simulink model "QuadrotorFinalProjectv4"  (R2018b)
settings: Solver=VariableStepAuto  StartTime=0.0  StopTime=25  RelTol=1e-3
undefined symbols (not defined in the file or in its folder): sigbuilder_block, X, Y, Z
libraries: sm_lib x94, nesl_utility x48, simulink x4
(part 3 of 3)

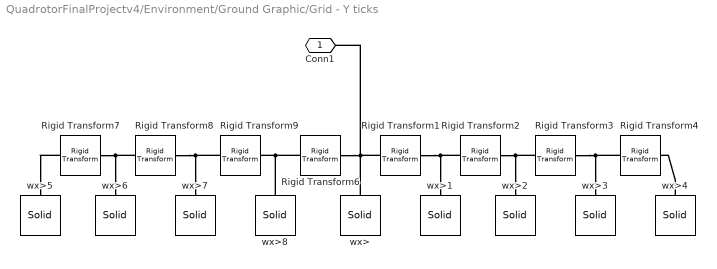
== system QuadrotorFinalProjectv4/Environment/Ground Graphic/Grid - Y ticks ==
  Rigid Transform{1..4,6..9} (8 alike) : sm_lib/Frames and Transforms/Rigid Transform  TranslationMethod=Cartesian  TranslationStandardOffset=0  TranslationLengthUnit=m  TranslationStandardAxis=+Z  TranslationCartesianOffset=[0 10 0]  TranslationROffset=0  TranslationROffsetUnits=m  TranslationZOffset=0  TranslationZOffsetUnits=m  TranslationThetaOffset=0  TranslationThetaOffsetUnits=deg  RotationMethod=None  RotationAngleUnits=deg  RotationStandardAxis=+Z  RotationAngle=0.0  RotationArbitraryAxis=[0 0 1]  FollAlignAxisA=+X  BaseAlignAxisA=+Y  FollAlignAxisB=+Y  BaseAlignAxisB=+Z  RotationSequenceAxes=FollowerAxes  RotationSequence=XYX  RotationSequenceAngles=[0 0 0]  RotationSequenceAnglesUnits=deg  RotationMatrix=[1 0 0; 0 1 0; 0 0 1]
  wx>{,1..8} (9 alike) : sm_lib/Body Elements/Solid  InertiaType=CalculateFromGeometry  Mass=1.6  MassUnits=kg  CenterOfMass=[0 0 0]  CenterOfMassUnits=m  MomentsOfInertia=[1 1 1]  MomentsOfInertiaUnits=kg*m^2  ProductsOfInertia=[0 0 0]  ProductsOfInertiaUnits=kg*m^2  BasedOnType=Mass  Density=1000  DensityUnits=kg/m^3  DoExposeReferenceFrame=on  SerializedFrames=<Frames/>  GraphicType=FromGeometry  MarkerShape=Frame  MarkerSize=10  GraphicVisPropType=SimpleVisualProperties  GraphicDiffuseColor=[1 1 1]  GraphicSpecularColor=[0.5 0.5 0.5 1.0]  GraphicAmbientColor=[0.15 0.15 0.15 1.0]  GraphicEmissiveColor=[0.0 0.0 0.0 1.0]  GraphicShininess=75  GraphicOpacity=0.9  GeometryShape=Brick  RectangleSize=[1 1]  RectangleSizeUnits=m  BrickDimensions=[100 1 0.12]  BrickDimensionUnits=m  CylinderRadius=1  CylinderRadiusUnits=m  CylinderLength=1  CylinderLengthUnits=m  SphereRadius=0.05  SphereRadiusUnits=m  EllipsoidRadii=[1 1 1]  EllipsoidRadiiUnits=m  ExtrusionCrossSection=[1 1; -1 1; -1 -1; 1 -1]  ExtrusionCrossSectionUnits=m  ExtrusionLength=1  ExtrusionLengthUnits=m  PolygonNumSides=3  PolygonOuterRadius=1  PolygonOuterRadiusUnits=m  ExtGeomFileType=STEP  ExtGeomFileUnits=m  RevolutionCrossSection=[1 1; 1 -1; 2 -1; 2 1]  RevolutionCrossSectionUnits=m  RevolutionExtent=Full  RevolutionAngle=180  RevolutionAngleUnits=deg
  Conn1 : PMIOPort  Side=Left
  connections:
  wx>/RConn1 -- Conn1/RConn1 -- Rigid Transform1/LConn1 -- Rigid Transform6/RConn1
  Rigid Transform2/LConn1 -- Rigid Transform1/RConn1 -- wx>1/RConn1
  Rigid Transform2/RConn1 -- Rigid Transform3/LConn1 -- wx>2/RConn1
  wx>8/RConn1 -- Rigid Transform6/LConn1 -- Rigid Transform9/RConn1
  wx>4/RConn1 -- Rigid Transform4/RConn1
  Rigid Transform7/RConn1 -- Rigid Transform8/LConn1 -- wx>6/RConn1
  Rigid Transform7/LConn1 -- wx>5/RConn1
  Rigid Transform3/RConn1 -- wx>3/RConn1 -- Rigid Transform4/LConn1
  Rigid Transform8/RConn1 -- Rigid Transform9/LConn1 -- wx>7/RConn1

== matlab function QuadrotorFinalProjectv4/Quadrotor/SmallSphere1Drag/MATLAB Function1 ==
  data: vx input; y output; vy input; vz input
function y = drag(vx,vy,vz)
radius = 0.02;
y = [-((1/2)*(1)*pi*(radius^(2))*(0.5)*(abs(vx))*vx); ...
    -((1/2)*(1)*pi*(radius^(2))*(0.5)*(abs(vy))*vy); ...
    -((1/2)*(1)*pi*(radius^(2))*(0.5)*(abs(vz))*vz)];

== matlab function QuadrotorFinalProjectv4/Quadrotor/LargeSphereDrag/MATLAB Function ==
  data: vx input; y output; vy input; vz input
function y = drag(vx,vy,vz)
radius = 0.05;
y = [-((1/2)*(1)*pi*(radius^(2))*(0.5)*(abs(vx))*vx); ...
    -((1/2)*(1)*pi*(radius^(2))*(0.5)*(abs(vy))*vy); ...
    -((1/2)*(1)*pi*(radius^(2))*(0.5)*(abs(vz))*vz)];

== matlab function QuadrotorFinalProjectv4/Quadrotor/SmallSphere2Drag/MATLAB Function1 ==
  data: vx input; y output; vy input; vz input
function y = drag(vx,vy,vz)
radius = 0.02;
y = [-((1/2)*(1)*pi*(radius^(2))*(0.5)*(abs(vx))*vx); ...
    -((1/2)*(1)*pi*(radius^(2))*(0.5)*(abs(vy))*vy); ...
    -((1/2)*(1)*pi*(radius^(2))*(0.5)*(abs(vz))*vz)];

== matlab function QuadrotorFinalProjectv4/Quadrotor/SmallSphere4Drag/MATLAB Function1 ==
  data: vx input; y output; vy input; vz input
function y = drag(vx,vy,vz)
radius = 0.02;
y = [-((1/2)*(1)*pi*(radius^(2))*(0.5)*(abs(vx))*vx); ...
    -((1/2)*(1)*pi*(radius^(2))*(0.5)*(abs(vy))*vy); ...
    -((1/2)*(1)*pi*(radius^(2))*(0.5)*(abs(vz))*vz)];

== matlab function QuadrotorFinalProjectv4/Quadrotor/SmallSphere3Drag/MATLAB Function1 ==
  data: vx input; y output; vy input; vz input
function y = drag(vx,vy,vz)
radius = 0.02;
y = [-((1/2)*(1)*pi*(radius^(2))*(0.5)*(abs(vx))*vx); ...
    -((1/2)*(1)*pi*(radius^(2))*(0.5)*(abs(vy))*vy); ...
    -((1/2)*(1)*pi*(radius^(2))*(0.5)*(abs(vz))*vz)];

== matlab function QuadrotorFinalProjectv4/MATLAB Function ==
  data: Fz input; t1 output; Mp input; Mq input; Mr input; t2 output; t3 output; t4 output
function [t1,t2,t3,t4] = calcTorque(Fz,Mp,Mq,Mr)

F = [Fz ; Mp ; Mq ; Mr];
A = [  1,  1,  1,  1; 
       1,  1, -1, -1;
      -1,  1,  1, -1;
      -1,  1, -1,  1];
T = linsolve(A,F);

t1 = .1+T(1,:);
t2 = .1+T(2,:);
t3 = .1+T(3,:);
t4 = .1+T(4,:);

== matlab function QuadrotorFinalProjectv4/getValues/MATLAB Function1 ==
  data: Q input; ang output
function ang = eulerAngles(Q)
e0= Q(1,:); e1= Q(2,:); e2= Q(3,:); e3= Q(4,:);
ang = quat2eul([e0 e1 e2 e3]);
